simulink model "test_8m_0508"  (R2024a)
settings: Solver=FixedStepAuto  StartTime=0.0  StopTime=30  FixedStep=dt  RelTol=1e-3
values from neighbouring files (symbols this model uses):
  attitude_0 = [0; -90;  -0]    [ini_param_8m_0522.m]
  b = 4.0    (= 4)    [ini_param_8m_0522.m]
  cbar = 0.75    [ini_param_8m_0522.m]
  dt = 0.004    [ini_param_8m_0522.m]
  H = 1000    [ini_param_8m_0522.m]
  N_data = [0,200, 491, 804, 1077, 1344, 1559, 1832, 2078, 2318, 2579,            2864, 3117, 3371, 3608.2, 3872, 4055.7, 4291, 4507, 4739, 4935]'    [cal_motor.m]
  N_pwm = 0.01*[0, 5 ,10 ,15 ,20 ,25 ,30 ,35,40, 45 ,50 ,              55 ,60 ,65 ,70, 75, 80 , 85 ,90 ,95 ,100]'    [cal_motor.m]
  pitch_rate_K = 1    [ini_param_8m_0522.m]
  roll_rate_K = 1    [ini_param_8m_0522.m]
  S = 6.0    (= 6)    [ini_param_8m_0522.m]
  Ts = 0.05    [ini_param_8m_0522.m]
  Ts_sur = 0.25    [ini_param_8m_0522.m]
  yaw_rate_K = 1    [ini_param_8m_0522.m]
undefined symbols (not defined in the file or in its folder): sigbuilder_block, UAV
libraries: slpidlib x9, simulink_extras x6, sharedtransform x2, shared6dof x1
(part 3 of 11)

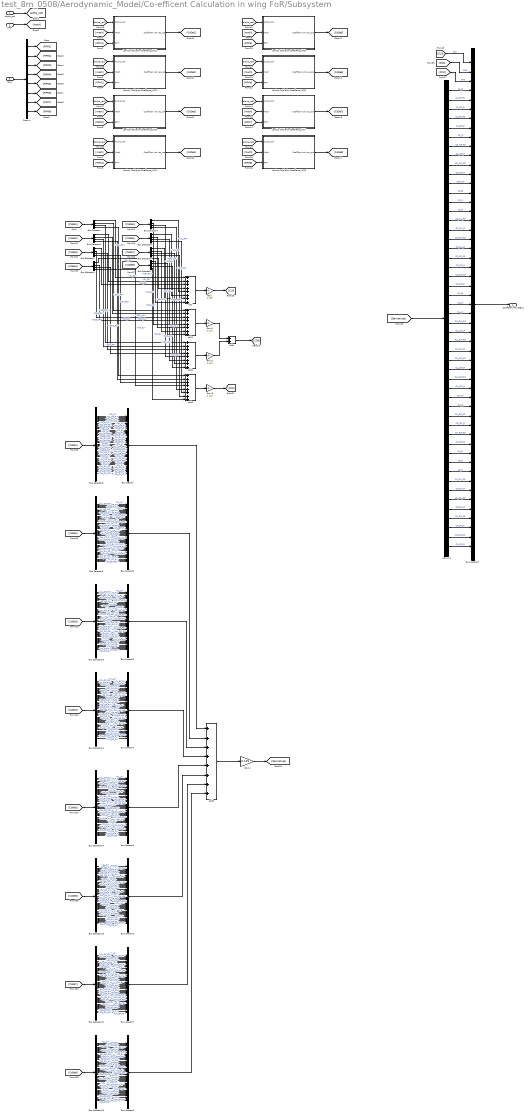
== system test_8m_0508/Aerodynamic_Model/Co-efficent Calculation in wing FoR/Subsystem ==
  alpha_rad : Inport
  Mach : Inport  Port=2
  RPM : Inport  Port=3
  Add{,1..3,5} (5 alike) : Sum  Inputs=++++++++
  Add4 : Sum
  Bus Creator{,2..8} (8 alike) : BusCreator  Inputs=50
  Bus Creator1 : BusCreator  Inputs=53
  Bus Selector : BusSelector  OutputSignals=CL_FR,CDI_FR,CD0_FR,CM_FR
  Bus Selector1 : BusSelector  OutputSignals=CL_FR,CDI_FR,CD0_FR,CM_FR
  Bus Selector{8..15} (8 alike) : BusSelector  OutputSignals=CL_Q,CL_DF_FO,CL_DF_FI,CL_DF_RO,CL_DF_RI,CD_Q,CD_DF_FO,CD_DF_FI,CD_DF_RO,CD_DF_RI,CD0_AF,CS_B,CS_P,CS_R,CS_DA_FO,CS_DA_FI,CS_DA_RO,CS_DA_RI,CS_DF_FO,CS_DF_FI,CS_DF_RO,CS_DF_RI,CLL_B,CLL_P,CLL_R,CLL_DA_FO,CLL_DA_FI,CLL_DA_RO,CLL_DA_RI,CLL_DF_FO,CLL_DF_FI,CLL_DF_RO,CLL_DF_RI,CM_AF,CM_Q,CM_DF_FO,CM_DF_FI,CM_DF_RO,CM_DF_RI,CN_B,CN_P,CN_R,CN_DA_FO,CN_DA_FI,CN_DA_RO,CN_DA_RI,CN_DF_FO,CN_DF_FI,CN_DF_RO,CN_DF_RI
  Bus Selector2 : BusSelector  OutputSignals=CL_FL,CDI_FL,CD0_FL,CM_FL
  Bus Selector3 : BusSelector  OutputSignals=CL_FL,CDI_FL,CD0_FL,CM_FL
  Bus Selector4 : BusSelector  OutputSignals=CL_RR,CDI_RR,CD0_RR,CM_RR
  Bus Selector5 : BusSelector  OutputSignals=CL_RR,CDI_RR,CD0_RR,CM_RR
  Bus Selector6 : BusSelector  OutputSignals=CL_RL,CDI_RL,CD0_RL,CM_RL
  Bus Selector7 : BusSelector  OutputSignals=CL_RL,CDI_RL,CD0_RL,CM_RL
  Demux : Demux  Outputs=8
  Demux1 : Demux  Outputs=50
  Gain{,1..4} (5 alike) : Gain  Gain=0.125
  LookUp Table for Coeffients_WS1 : Subsystem
  LookUp Table for Coeffients_WS2 : Subsystem
  LookUp Table for Coeffients_WS3 : Subsystem
  LookUp Table for Coeffients_WS4 : Subsystem
  LookUp Table for Coeffients_WS5 : Subsystem
  LookUp Table for Coeffients_WS6 : Subsystem
  LookUp Table for Coeffients_WS7 : Subsystem
  LookUp Table for Coeffients_WS8 : Subsystem
  CoeffDerivativesBus : Outport
  wires:
  [alpha_rad] -> LookUp Table for Coeffients_WS6/1(alpha_rad)
  [alpha_rad] -> LookUp Table for Coeffients_WS5/1(alpha_rad)
  [alpha_rad] -> LookUp Table for Coeffients_WS7/1(alpha_rad)
  [alpha_rad] -> LookUp Table for Coeffients_WS4/1(alpha_rad)
  [alpha_rad] -> LookUp Table for Coeffients_WS8/1(alpha_rad)
  [alpha_rad] -> LookUp Table for Coeffients_WS3/1(alpha_rad)
  [alpha_rad] -> LookUp Table for Coeffients_WS2/1(alpha_rad)
  [alpha_rad] -> LookUp Table for Coeffients_WS1/1(alpha_rad)
  RPM/1 -> Demux/1
  Demux/1 -> [RPM1]
  alpha_rad/1 -> [alpha_rad]
  Mach/1 -> [mach]
  Demux/2 -> [RPM2]
  Demux/3 -> [RPM3]
  Demux/4 -> [RPM4]
  Demux/5 -> [RPM5]
  Demux/6 -> [RPM6]
  Demux/7 -> [RPM7]
  Demux/8 -> [RPM8]
  [mach] -> LookUp Table for Coeffients_WS1/2(Mach)
  [RPM1] -> LookUp Table for Coeffients_WS1/3(RPM)
  [mach] -> LookUp Table for Coeffients_WS2/2(Mach)
  [RPM2] -> LookUp Table for Coeffients_WS2/3(RPM)
  [mach] -> LookUp Table for Coeffients_WS3/2(Mach)
  [RPM3] -> LookUp Table for Coeffients_WS3/3(RPM)
  [mach] -> LookUp Table for Coeffients_WS4/2(Mach)
  [RPM4] -> LookUp Table for Coeffients_WS4/3(RPM)
  [mach] -> LookUp Table for Coeffients_WS5/2(Mach)
  [RPM5] -> LookUp Table for Coeffients_WS5/3(RPM)
  [mach] -> LookUp Table for Coeffients_WS6/2(Mach)
  [RPM6] -> LookUp Table for Coeffients_WS6/3(RPM)
  [mach] -> LookUp Table for Coeffients_WS7/2(Mach)
  [RPM7] -> LookUp Table for Coeffients_WS7/3(RPM)
  [mach] -> LookUp Table for Coeffients_WS8/2(Mach)
  [RPM8] -> LookUp Table for Coeffients_WS8/3(RPM)
  LookUp Table for Coeffients_WS1/1(CoeffDerivatives_rad) -> [CoDe1]
  LookUp Table for Coeffients_WS2/1(CoeffDerivatives_rad) -> [CoDe2]
  LookUp Table for Coeffients_WS3/1(CoeffDerivatives_rad) -> [CoDe3]
  LookUp Table for Coeffients_WS4/1(CoeffDerivatives_rad) -> [CoDe4]
  LookUp Table for Coeffients_WS5/1(CoeffDerivatives_rad) -> [CoDe5]
  LookUp Table for Coeffients_WS6/1(CoeffDerivatives_rad) -> [CoDe6]
  LookUp Table for Coeffients_WS7/1(CoeffDerivatives_rad) -> [CoDe7]
  LookUp Table for Coeffients_WS8/1(CoeffDerivatives_rad) -> [CoDe8]
  Bus Creator1/1 -> CoeffDerivativesBus/1
  [CoDe1] -> Bus Selector/1
  [CoDe7] -> Bus Selector6/1
  [CoDe5] -> Bus Selector4/1
  [CoDe3] -> Bus Selector2/1
  [CoDe4] -> Bus Selector3/1
  [CoDe2] -> Bus Selector1/1
  [CoDe6] -> Bus Selector5/1
  [CoDe8] -> Bus Selector7/1
  Bus Selector/1 -> Add/1  "<CL_FR>"
  Bus Selector1/1 -> Add/2  "<CL_FR>"
  Bus Selector2/1 -> Add/3  "<CL_FL>"
  Bus Selector3/1 -> Add/4  "<CL_FL>"
  Bus Selector4/1 -> Add/5  "<CL_RR>"
  Bus Selector5/1 -> Add/6  "<CL_RR>"
  Bus Selector6/1 -> Add/7  "<CL_RL>"
  Bus Selector7/1 -> Add/8  "<CL_RL>"
  Add/1 -> Gain/1
  Add1/1 -> Gain1/1
  Add2/1 -> Gain2/1
  Add3/1 -> Gain3/1
  Bus Selector/2 -> Add1/1  "<CDI_FR>"
  Bus Selector1/2 -> Add1/2  "<CDI_FR>"
  Bus Selector2/2 -> Add1/3  "<CDI_FL>"
  Bus Selector3/2 -> Add1/4  "<CDI_FL>"
  Bus Selector4/2 -> Add1/5  "<CDI_RR>"
  Bus Selector5/2 -> Add1/6  "<CDI_RR>"
  Bus Selector6/2 -> Add1/7  "<CDI_RL>"
  Bus Selector7/2 -> Add1/8  "<CDI_RL>"
  Bus Selector/3 -> Add2/1  "<CD0_FR>"
  Bus Selector1/3 -> Add2/2  "<CD0_FR>"
  Bus Selector2/3 -> Add2/3  "<CD0_FL>"
  Bus Selector3/3 -> Add2/4  "<CD0_FL>"
  Bus Selector4/3 -> Add2/5  "<CD0_RR>"
  Bus Selector5/3 -> Add2/6  "<CD0_RR>"
  Bus Selector6/3 -> Add2/7  "<CD0_RL>"
  Bus Selector7/3 -> Add2/8  "<CD0_RL>"
  Bus Selector/4 -> Add3/1  "<CM_FR>"
  Bus Selector1/4 -> Add3/2  "<CM_FR>"
  Bus Selector2/4 -> Add3/3  "<CM_FL>"
  Bus Selector3/4 -> Add3/4  "<CM_FL>"
  Bus Selector4/4 -> Add3/5  "<CM_RR>"
  Bus Selector5/4 -> Add3/6  "<CM_RR>"
  Bus Selector6/4 -> Add3/7  "<CM_RL>"
  Bus Selector7/4 -> Add3/8  "<CM_RL>"
  Gain/1 -> [CL0]
  Gain1/1 -> Add4/1
  Gain2/1 -> Add4/2
  Gain3/1 -> [CM0]
  Add4/1 -> [CD0]
  [CoDe1] -> Bus Selector8/1
  Bus Selector8/1 -> Bus Creator/1  "<CL_Q>"
  Bus Selector8/2 -> Bus Creator/2  "<CL_DF_FO>"
  Bus Selector8/3 -> Bus Creator/3  "<CL_DF_FI>"
  Bus Selector8/4 -> Bus Creator/4  "<CL_DF_RO>"
  Bus Selector8/5 -> Bus Creator/5  "<CL_DF_RI>"
  Bus Selector8/6 -> Bus Creator/6  "<CD_Q>"
  Bus Selector8/7 -> Bus Creator/7  "<CD_DF_FO>"
  Bus Selector8/8 -> Bus Creator/8  "<CD_DF_FI>"
  Bus Selector8/9 -> Bus Creator/9  "<CD_DF_RO>"
  Bus Selector8/10 -> Bus Creator/10  "<CD_DF_RI>"
  Bus Selector8/11 -> Bus Creator/11  "<CD0_AF>"
  Bus Selector8/12 -> Bus Creator/12  "<CS_B>"
  Bus Selector8/13 -> Bus Creator/13  "<CS_P>"
  Bus Selector8/14 -> Bus Creator/14  "<CS_R>"
  Bus Selector8/15 -> Bus Creator/15  "<CS_DA_FO>"
  Bus Selector8/16 -> Bus Creator/16  "<CS_DA_FI>"
  Bus Selector8/17 -> Bus Creator/17  "<CS_DA_RO>"
  Bus Selector8/18 -> Bus Creator/18  "<CS_DA_RI>"
  Bus Selector8/19 -> Bus Creator/19  "<CS_DF_FO>"
  Bus Selector8/20 -> Bus Creator/20  "<CS_DF_FI>"
  Bus Selector8/21 -> Bus Creator/21  "<CS_DF_RO>"
  Bus Selector8/22 -> Bus Creator/22  "<CS_DF_RI>"
  Bus Selector8/23 -> Bus Creator/23  "<CLL_B>"
  Bus Selector8/24 -> Bus Creator/24  "<CLL_P>"
  Bus Selector8/25 -> Bus Creator/25  "<CLL_R>"
  Bus Selector8/26 -> Bus Creator/26  "<CLL_DA_FO>"
  Bus Selector8/27 -> Bus Creator/27  "<CLL_DA_FI>"
  Bus Selector8/28 -> Bus Creator/28  "<CLL_DA_RO>"
  Bus Selector8/29 -> Bus Creator/29  "<CLL_DA_RI>"
  Bus Selector8/30 -> Bus Creator/30  "<CLL_DF_FO>"
  Bus Selector8/31 -> Bus Creator/31  "<CLL_DF_FI>"
  Bus Selector8/32 -> Bus Creator/32  "<CLL_DF_RO>"
  Bus Selector8/33 -> Bus Creator/33  "<CLL_DF_RI>"
  Bus Selector8/34 -> Bus Creator/34  "<CM_AF>"
  Bus Selector8/35 -> Bus Creator/35  "<CM_Q>"
  Bus Selector8/36 -> Bus Creator/36  "<CM_DF_FO>"
  Bus Selector8/37 -> Bus Creator/37  "<CM_DF_FI>"
  Bus Selector8/38 -> Bus Creator/38  "<CM_DF_RO>"
  Bus Selector8/39 -> Bus Creator/39  "<CM_DF_RI>"
  Bus Selector8/40 -> Bus Creator/40  "<CN_B>"
  Bus Selector8/41 -> Bus Creator/41  "<CN_P>"
  Bus Selector8/42 -> Bus Creator/42  "<CN_R>"
  Bus Selector8/43 -> Bus Creator/43  "<CN_DA_FO>"
  Bus Selector8/44 -> Bus Creator/44  "<CN_DA_FI>"
  Bus Selector8/45 -> Bus Creator/45  "<CN_DA_RO>"
  Bus Selector8/46 -> Bus Creator/46  "<CN_DA_RI>"
  Bus Selector8/47 -> Bus Creator/47  "<CN_DF_FO>"
  Bus Selector8/48 -> Bus Creator/48  "<CN_DF_FI>"
  Bus Selector8/49 -> Bus Creator/49  "<CN_DF_RO>"
  Bus Selector8/50 -> Bus Creator/50  "<CN_DF_RI>"
  Bus Selector9/21 -> Bus Creator2/21  "<CS_DF_RO>"
  Bus Selector9/26 -> Bus Creator2/26  "<CLL_DA_FO>"
  Bus Selector9/19 -> Bus Creator2/19  "<CS_DF_FO>"
  Bus Selector9/22 -> Bus Creator2/22  "<CS_DF_RI>"
  Bus Selector9/16 -> Bus Creator2/16  "<CS_DA_FI>"
  Bus Selector9/13 -> Bus Creator2/13  "<CS_P>"
  Bus Selector9/17 -> Bus Creator2/17  "<CS_DA_RO>"
  Bus Selector9/14 -> Bus Creator2/14  "<CS_R>"
  Bus Selector9/15 -> Bus Creator2/15  "<CS_DA_FO>"
  Bus Selector9/12 -> Bus Creator2/12  "<CS_B>"
  Bus Selector9/18 -> Bus Creator2/18  "<CS_DA_RI>"
  Bus Selector9/8 -> Bus Creator2/8  "<CD_DF_FI>"
  Bus Selector9/7 -> Bus Creator2/7  "<CD_DF_FO>"
  Bus Selector9/9 -> Bus Creator2/9  "<CD_DF_RO>"
  Bus Selector9/3 -> Bus Creator2/3  "<CL_DF_FI>"
  Bus Selector9/4 -> Bus Creator2/4  "<CL_DF_RO>"
  Bus Selector9/5 -> Bus Creator2/5  "<CL_DF_RI>"
  Bus Selector9/28 -> Bus Creator2/28  "<CLL_DA_RO>"
  [CoDe2] -> Bus Selector9/1
  Bus Selector9/40 -> Bus Creator2/40  "<CN_B>"
  Bus Selector9/27 -> Bus Creator2/27  "<CLL_DA_FI>"
  Bus Selector9/39 -> Bus Creator2/39  "<CM_DF_RI>"
  Bus Selector9/24 -> Bus Creator2/24  "<CLL_P>"
  Bus Selector9/33 -> Bus Creator2/33  "<CLL_DF_RI>"
  Bus Selector9/31 -> Bus Creator2/31  "<CLL_DF_FI>"
  Bus Selector9/32 -> Bus Creator2/32  "<CLL_DF_RO>"
  Bus Selector9/37 -> Bus Creator2/37  "<CM_DF_FI>"
  Bus Selector9/35 -> Bus Creator2/35  "<CM_Q>"
  Bus Selector9/34 -> Bus Creator2/34  "<CM_AF>"
  Bus Selector9/38 -> Bus Creator2/38  "<CM_DF_RO>"
  Bus Selector9/11 -> Bus Creator2/11  "<CD0_AF>"
  Bus Selector9/36 -> Bus Creator2/36  "<CM_DF_FO>"
  Bus Selector9/30 -> Bus Creator2/30  "<CLL_DF_FO>"
  Bus Selector9/29 -> Bus Creator2/29  "<CLL_DA_RI>"
  Bus Selector9/6 -> Bus Creator2/6  "<CD_Q>"
  Bus Selector9/49 -> Bus Creator2/49  "<CN_DF_RO>"
  Bus Selector9/23 -> Bus Creator2/23  "<CLL_B>"
  Bus Selector9/50 -> Bus Creator2/50  "<CN_DF_RI>"
  Bus Selector9/20 -> Bus Creator2/20  "<CS_DF_FI>"
  Bus Selector9/48 -> Bus Creator2/48  "<CN_DF_FI>"
  Bus Selector9/47 -> Bus Creator2/47  "<CN_DF_FO>"
  Bus Selector9/44 -> Bus Creator2/44  "<CN_DA_FI>"
  Bus Selector9/42 -> Bus Creator2/42  "<CN_R>"
  Bus Selector9/10 -> Bus Creator2/10  "<CD_DF_RI>"
  Bus Selector9/25 -> Bus Creator2/25  "<CLL_R>"
  Bus Selector9/45 -> Bus Creator2/45  "<CN_DA_RO>"
  Bus Selector9/43 -> Bus Creator2/43  "<CN_DA_FO>"
  Bus Selector9/46 -> Bus Creator2/46  "<CN_DA_RI>"
  Bus Selector9/2 -> Bus Creator2/2  "<CL_DF_FO>"
  Bus Selector9/41 -> Bus Creator2/41  "<CN_P>"
  Bus Selector9/1 -> Bus Creator2/1  "<CL_Q>"
  Bus Selector11/9 -> Bus Creator4/9  "<CD_DF_RO>"
  Bus Selector11/7 -> Bus Creator4/7  "<CD_DF_FO>"
  Bus Selector11/14 -> Bus Creator4/14  "<CS_R>"
  Bus Selector11/17 -> Bus Creator4/17  "<CS_DA_RO>"
  Bus Selector11/8 -> Bus Creator4/8  "<CD_DF_FI>"
  Bus Selector11/12 -> Bus Creator4/12  "<CS_B>"
  Bus Selector11/15 -> Bus Creator4/15  "<CS_DA_FO>"
  Bus Selector11/19 -> Bus Creator4/19  "<CS_DF_FO>"
  Bus Selector11/26 -> Bus Creator4/26  "<CLL_DA_FO>"
  Bus Selector11/13 -> Bus Creator4/13  "<CS_P>"
  Bus Selector11/16 -> Bus Creator4/16  "<CS_DA_FI>"
  Bus Selector11/21 -> Bus Creator4/21  "<CS_DF_RO>"
  Bus Selector10/28 -> Bus Creator3/28  "<CLL_DA_RO>"
  Bus Selector10/27 -> Bus Creator3/27  "<CLL_DA_FI>"
  Bus Selector10/23 -> Bus Creator3/23  "<CLL_B>"
  Bus Selector10/25 -> Bus Creator3/25  "<CLL_R>"
  Bus Selector10/20 -> Bus Creator3/20  "<CS_DF_FI>"
  Bus Selector10/21 -> Bus Creator3/21  "<CS_DF_RO>"
  Bus Selector10/26 -> Bus Creator3/26  "<CLL_DA_FO>"
  Bus Selector10/24 -> Bus Creator3/24  "<CLL_P>"
  Bus Selector10/19 -> Bus Creator3/19  "<CS_DF_FO>"
  Bus Selector10/22 -> Bus Creator3/22  "<CS_DF_RI>"
  Bus Selector10/16 -> Bus Creator3/16  "<CS_DA_FI>"
  Bus Selector10/13 -> Bus Creator3/13  "<CS_P>"
  Bus Selector10/17 -> Bus Creator3/17  "<CS_DA_RO>"
  Bus Selector10/14 -> Bus Creator3/14  "<CS_R>"
  Bus Selector10/15 -> Bus Creator3/15  "<CS_DA_FO>"
  Bus Selector10/11 -> Bus Creator3/11  "<CD0_AF>"
  Bus Selector10/10 -> Bus Creator3/10  "<CD_DF_RI>"
  Bus Selector10/12 -> Bus Creator3/12  "<CS_B>"
  Bus Selector10/18 -> Bus Creator3/18  "<CS_DA_RI>"
  Bus Selector10/8 -> Bus Creator3/8  "<CD_DF_FI>"
  Bus Selector10/7 -> Bus Creator3/7  "<CD_DF_FO>"
  Bus Selector10/9 -> Bus Creator3/9  "<CD_DF_RO>"
  Bus Selector10/3 -> Bus Creator3/3  "<CL_DF_FI>"
  Bus Selector10/4 -> Bus Creator3/4  "<CL_DF_RO>"
  [CoDe3] -> Bus Selector10/1
  Bus Selector10/39 -> Bus Creator3/39  "<CM_DF_RI>"
  Bus Selector10/37 -> Bus Creator3/37  "<CM_DF_FI>"
  Bus Selector10/34 -> Bus Creator3/34  "<CM_AF>"
  Bus Selector10/38 -> Bus Creator3/38  "<CM_DF_RO>"
  Bus Selector10/36 -> Bus Creator3/36  "<CM_DF_FO>"
  Bus Selector10/49 -> Bus Creator3/49  "<CN_DF_RO>"
  Bus Selector10/45 -> Bus Creator3/45  "<CN_DA_RO>"
  Bus Selector10/46 -> Bus Creator3/46  "<CN_DA_RI>"
  Bus Selector10/42 -> Bus Creator3/42  "<CN_R>"
  Bus Selector10/41 -> Bus Creator3/41  "<CN_P>"
  Bus Selector10/43 -> Bus Creator3/43  "<CN_DA_FO>"
  Bus Selector10/29 -> Bus Creator3/29  "<CLL_DA_RI>"
  Bus Selector10/6 -> Bus Creator3/6  "<CD_Q>"
  Bus Selector11/1 -> Bus Creator4/1  "<CL_Q>"
  Bus Selector11/46 -> Bus Creator4/46  "<CN_DA_RI>"
  Bus Selector10/2 -> Bus Creator3/2  "<CL_DF_FO>"
  Bus Selector10/31 -> Bus Creator3/31  "<CLL_DF_FI>"
  Bus Selector11/41 -> Bus Creator4/41  "<CN_P>"
  Bus Selector11/25 -> Bus Creator4/25  "<CLL_R>"
  Bus Selector11/45 -> Bus Creator4/45  "<CN_DA_RO>"
  Bus Selector11/10 -> Bus Creator4/10  "<CD_DF_RI>"
  Bus Selector11/18 -> Bus Creator4/18  "<CS_DA_RI>"
  Bus Selector11/42 -> Bus Creator4/42  "<CN_R>"
  Bus Selector11/50 -> Bus Creator4/50  "<CN_DF_RI>"
  Bus Selector10/47 -> Bus Creator3/47  "<CN_DF_FO>"
  Bus Selector11/23 -> Bus Creator4/23  "<CLL_B>"
  Bus Selector11/48 -> Bus Creator4/48  "<CN_DF_FI>"
  Bus Selector11/20 -> Bus Creator4/20  "<CS_DF_FI>"
  Bus Selector10/50 -> Bus Creator3/50  "<CN_DF_RI>"
  Bus Selector11/6 -> Bus Creator4/6  "<CD_Q>"
  Bus Selector11/47 -> Bus Creator4/47  "<CN_DF_FO>"
  Bus Selector11/11 -> Bus Creator4/11  "<CD0_AF>"
  Bus Selector11/38 -> Bus Creator4/38  "<CM_DF_RO>"
  Bus Selector10/33 -> Bus Creator3/33  "<CLL_DF_RI>"
  Bus Selector11/30 -> Bus Creator4/30  "<CLL_DF_FO>"
  Bus Selector11/36 -> Bus Creator4/36  "<CM_DF_FO>"
  Bus Selector11/22 -> Bus Creator4/22  "<CS_DF_RI>"
  Bus Selector10/44 -> Bus Creator3/44  "<CN_DA_FI>"
  Bus Selector11/35 -> Bus Creator4/35  "<CM_Q>"
  Bus Selector10/35 -> Bus Creator3/35  "<CM_Q>"
  Bus Selector11/34 -> Bus Creator4/34  "<CM_AF>"
  Bus Selector10/32 -> Bus Creator3/32  "<CLL_DF_RO>"
  Bus Selector11/31 -> Bus Creator4/31  "<CLL_DF_FI>"
  Bus Selector11/2 -> Bus Creator4/2  "<CL_DF_FO>"
  Bus Selector11/40 -> Bus Creator4/40  "<CN_B>"
  Bus Selector11/24 -> Bus Creator4/24  "<CLL_P>"
  Bus Selector11/43 -> Bus Creator4/43  "<CN_DA_FO>"
  Bus Selector11/27 -> Bus Creator4/27  "<CLL_DA_FI>"
  Bus Selector10/30 -> Bus Creator3/30  "<CLL_DF_FO>"
  Bus Selector11/3 -> Bus Creator4/3  "<CL_DF_FI>"
  Bus Selector10/40 -> Bus Creator3/40  "<CN_B>"
  Bus Selector11/37 -> Bus Creator4/37  "<CM_DF_FI>"
  Bus Selector11/29 -> Bus Creator4/29  "<CLL_DA_RI>"
  Bus Selector11/5 -> Bus Creator4/5  "<CL_DF_RI>"
  [CoDe4] -> Bus Selector11/1
  Bus Selector11/33 -> Bus Creator4/33  "<CLL_DF_RI>"
  Bus Selector11/44 -> Bus Creator4/44  "<CN_DA_FI>"
  Bus Selector11/4 -> Bus Creator4/4  "<CL_DF_RO>"
  Bus Selector11/49 -> Bus Creator4/49  "<CN_DF_RO>"
  Bus Selector10/48 -> Bus Creator3/48  "<CN_DF_FI>"
  Bus Selector11/28 -> Bus Creator4/28  "<CLL_DA_RO>"
  Bus Selector10/1 -> Bus Creator3/1  "<CL_Q>"
  Bus Selector11/32 -> Bus Creator4/32  "<CLL_DF_RO>"
  Bus Selector11/39 -> Bus Creator4/39  "<CM_DF_RI>"
  Bus Selector10/5 -> Bus Creator3/5  "<CL_DF_RI>"
  Bus Selector12/19 -> Bus Creator7/19  "<CS_DF_FO>"
  Bus Selector12/22 -> Bus Creator7/22  "<CS_DF_RI>"
  Bus Selector12/27 -> Bus Creator7/27  "<CLL_DA_FI>"
  Bus Selector12/21 -> Bus Creator7/21  "<CS_DF_RO>"
  Bus Selector13/21 -> Bus Creator8/21  "<CS_DF_RO>"
  Bus Selector12/20 -> Bus Creator7/20  "<CS_DF_FI>"
  Bus Selector12/26 -> Bus Creator7/26  "<CLL_DA_FO>"
  Bus Selector12/25 -> Bus Creator7/25  "<CLL_R>"
  Bus Selector13/8 -> Bus Creator8/8  "<CD_DF_FI>"
  Bus Selector13/19 -> Bus Creator8/19  "<CS_DF_FO>"
  Bus Selector13/17 -> Bus Creator8/17  "<CS_DA_RO>"
  Bus Selector13/7 -> Bus Creator8/7  "<CD_DF_FO>"
  Bus Selector13/26 -> Bus Creator8/26  "<CLL_DA_FO>"
  Bus Selector13/13 -> Bus Creator8/13  "<CS_P>"
  Bus Selector13/9 -> Bus Creator8/9  "<CD_DF_RO>"
  Bus Selector15/9 -> Bus Creator6/9  "<CD_DF_RO>"
  Bus Selector15/7 -> Bus Creator6/7  "<CD_DF_FO>"
  Bus Selector15/14 -> Bus Creator6/14  "<CS_R>"
  Bus Selector12/24 -> Bus Creator7/24  "<CLL_P>"
  Bus Selector15/17 -> Bus Creator6/17  "<CS_DA_RO>"
  Bus Selector15/12 -> Bus Creator6/12  "<CS_B>"
  Bus Selector15/15 -> Bus Creator6/15  "<CS_DA_FO>"
  Bus Selector15/19 -> Bus Creator6/19  "<CS_DF_FO>"
  Bus Selector15/26 -> Bus Creator6/26  "<CLL_DA_FO>"
  Bus Selector15/13 -> Bus Creator6/13  "<CS_P>"
  Bus Selector15/16 -> Bus Creator6/16  "<CS_DA_FI>"
  Bus Selector15/21 -> Bus Creator6/21  "<CS_DF_RO>"
  Bus Selector14/28 -> Bus Creator5/28  "<CLL_DA_RO>"
  Bus Selector14/27 -> Bus Creator5/27  "<CLL_DA_FI>"
  Bus Selector14/23 -> Bus Creator5/23  "<CLL_B>"
  Bus Selector14/25 -> Bus Creator5/25  "<CLL_R>"
  Bus Selector14/26 -> Bus Creator5/26  "<CLL_DA_FO>"
  Bus Selector14/24 -> Bus Creator5/24  "<CLL_P>"
  Bus Selector14/19 -> Bus Creator5/19  "<CS_DF_FO>"
  Bus Selector14/22 -> Bus Creator5/22  "<CS_DF_RI>"
  Bus Selector14/16 -> Bus Creator5/16  "<CS_DA_FI>"
  Bus Selector14/13 -> Bus Creator5/13  "<CS_P>"
  Bus Selector14/15 -> Bus Creator5/15  "<CS_DA_FO>"
  Bus Selector14/11 -> Bus Creator5/11  "<CD0_AF>"
  Bus Selector14/10 -> Bus Creator5/10  "<CD_DF_RI>"
  Bus Selector14/12 -> Bus Creator5/12  "<CS_B>"
  Bus Selector14/18 -> Bus Creator5/18  "<CS_DA_RI>"
  Bus Selector14/8 -> Bus Creator5/8  "<CD_DF_FI>"
  Bus Selector14/7 -> Bus Creator5/7  "<CD_DF_FO>"
  Bus Selector14/9 -> Bus Creator5/9  "<CD_DF_RO>"
  Bus Selector14/3 -> Bus Creator5/3  "<CL_DF_FI>"
  Bus Selector13/15 -> Bus Creator8/15  "<CS_DA_FO>"
  Bus Selector14/4 -> Bus Creator5/4  "<CL_DF_RO>"
  Bus Selector14/5 -> Bus Creator5/5  "<CL_DF_RI>"
  Bus Selector12/1 -> Bus Creator7/1  "<CL_Q>"
  Bus Selector13/32 -> Bus Creator8/32  "<CLL_DF_RO>"
  Bus Selector14/17 -> Bus Creator5/17  "<CS_DA_RO>"
  Bus Selector12/5 -> Bus Creator7/5  "<CL_DF_RI>"
  Bus Selector13/49 -> Bus Creator8/49  "<CN_DF_RO>"
  Bus Selector13/4 -> Bus Creator8/4  "<CL_DF_RO>"
  Bus Selector13/33 -> Bus Creator8/33  "<CLL_DF_RI>"
  Bus Selector12/30 -> Bus Creator7/30  "<CLL_DF_FO>"
  Bus Selector13/5 -> Bus Creator8/5  "<CL_DF_RI>"
  Bus Selector14/20 -> Bus Creator5/20  "<CS_DF_FI>"
  [CoDe8] -> Bus Selector13/1
  Bus Selector14/21 -> Bus Creator5/21  "<CS_DF_RO>"
  Bus Selector12/40 -> Bus Creator7/40  "<CN_B>"
  Bus Selector13/37 -> Bus Creator8/37  "<CM_DF_FI>"
  Bus Selector13/3 -> Bus Creator8/3  "<CL_DF_FI>"
  Bus Selector13/44 -> Bus Creator8/44  "<CN_DA_FI>"
  Bus Selector13/24 -> Bus Creator8/24  "<CLL_P>"
  Bus Selector13/2 -> Bus Creator8/2  "<CL_DF_FO>"
  Bus Selector13/40 -> Bus Creator8/40  "<CN_B>"
  Bus Selector13/27 -> Bus Creator8/27  "<CLL_DA_FI>"
  Bus Selector13/31 -> Bus Creator8/31  "<CLL_DF_FI>"
  Bus Selector12/32 -> Bus Creator7/32  "<CLL_DF_RO>"
  Bus Selector13/34 -> Bus Creator8/34  "<CM_AF>"
  Bus Selector13/35 -> Bus Creator8/35  "<CM_Q>"
  Bus Selector12/35 -> Bus Creator7/35  "<CM_Q>"
  [CoDe5] -> Bus Selector14/1
  Bus Selector14/40 -> Bus Creator5/40  "<CN_B>"
  Bus Selector14/39 -> Bus Creator5/39  "<CM_DF_RI>"
  Bus Selector14/38 -> Bus Creator5/38  "<CM_DF_RO>"
  Bus Selector14/33 -> Bus Creator5/33  "<CLL_DF_RI>"
  Bus Selector14/32 -> Bus Creator5/32  "<CLL_DF_RO>"
  Bus Selector14/37 -> Bus Creator5/37  "<CM_DF_FI>"
  Bus Selector14/35 -> Bus Creator5/35  "<CM_Q>"
  Bus Selector14/34 -> Bus Creator5/34  "<CM_AF>"
  Bus Selector14/36 -> Bus Creator5/36  "<CM_DF_FO>"
  Bus Selector14/30 -> Bus Creator5/30  "<CLL_DF_FO>"
  Bus Selector14/29 -> Bus Creator5/29  "<CLL_DA_RI>"
  Bus Selector14/49 -> Bus Creator5/49  "<CN_DF_RO>"
  Bus Selector14/50 -> Bus Creator5/50  "<CN_DF_RI>"
  Bus Selector14/48 -> Bus Creator5/48  "<CN_DF_FI>"
  Bus Selector14/47 -> Bus Creator5/47  "<CN_DF_FO>"
  Bus Selector14/45 -> Bus Creator5/45  "<CN_DA_RO>"
  Bus Selector14/46 -> Bus Creator5/46  "<CN_DA_RI>"
  Bus Selector14/44 -> Bus Creator5/44  "<CN_DA_FI>"
  Bus Selector14/42 -> Bus Creator5/42  "<CN_R>"
  Bus Selector14/41 -> Bus Creator5/41  "<CN_P>"
  Bus Selector14/43 -> Bus Creator5/43  "<CN_DA_FO>"
  Bus Selector14/2 -> Bus Creator5/2  "<CL_DF_FO>"
  Bus Selector15/2 -> Bus Creator6/2  "<CL_DF_FO>"
  Bus Selector12/28 -> Bus Creator7/28  "<CLL_DA_RO>"
  Bus Selector15/43 -> Bus Creator6/43  "<CN_DA_FO>"
  Bus Selector15/46 -> Bus Creator6/46  "<CN_DA_RI>"
  Bus Selector15/41 -> Bus Creator6/41  "<CN_P>"
  Bus Selector14/31 -> Bus Creator5/31  "<CLL_DF_FI>"
  Bus Selector13/29 -> Bus Creator8/29  "<CLL_DA_RI>"
  Bus Selector15/45 -> Bus Creator6/45  "<CN_DA_RO>"
  Bus Selector15/44 -> Bus Creator6/44  "<CN_DA_FI>"
  Bus Selector15/25 -> Bus Creator6/25  "<CLL_R>"
  Bus Selector15/10 -> Bus Creator6/10  "<CD_DF_RI>"
  Bus Selector15/18 -> Bus Creator6/18  "<CS_DA_RI>"
  Bus Selector15/50 -> Bus Creator6/50  "<CN_DF_RI>"
  Bus Selector15/23 -> Bus Creator6/23  "<CLL_B>"
  Bus Selector15/20 -> Bus Creator6/20  "<CS_DF_FI>"
  Bus Selector15/49 -> Bus Creator6/49  "<CN_DF_RO>"
  Bus Selector12/23 -> Bus Creator7/23  "<CLL_B>"
  Bus Selector15/6 -> Bus Creator6/6  "<CD_Q>"
  Bus Selector15/11 -> Bus Creator6/11  "<CD0_AF>"
  Bus Selector15/47 -> Bus Creator6/47  "<CN_DF_FO>"
  Bus Selector15/38 -> Bus Creator6/38  "<CM_DF_RO>"
  Bus Selector15/30 -> Bus Creator6/30  "<CLL_DF_FO>"
  Bus Selector15/36 -> Bus Creator6/36  "<CM_DF_FO>"
  Bus Selector15/22 -> Bus Creator6/22  "<CS_DF_RI>"
  Bus Selector15/35 -> Bus Creator6/35  "<CM_Q>"
  Bus Selector13/12 -> Bus Creator8/12  "<CS_B>"
  Bus Selector15/34 -> Bus Creator6/34  "<CM_AF>"
  Bus Selector15/37 -> Bus Creator6/37  "<CM_DF_FI>"
  Bus Selector13/39 -> Bus Creator8/39  "<CM_DF_RI>"
  Bus Selector15/31 -> Bus Creator6/31  "<CLL_DF_FI>"
  Bus Selector15/32 -> Bus Creator6/32  "<CLL_DF_RO>"
  Bus Selector15/24 -> Bus Creator6/24  "<CLL_P>"
  Bus Selector15/27 -> Bus Creator6/27  "<CLL_DA_FI>"
  Bus Selector15/3 -> Bus Creator6/3  "<CL_DF_FI>"
  Bus Selector15/4 -> Bus Creator6/4  "<CL_DF_RO>"
  Bus Selector13/43 -> Bus Creator8/43  "<CN_DA_FO>"
  Bus Selector12/2 -> Bus Creator7/2  "<CL_DF_FO>"
  Bus Selector13/14 -> Bus Creator8/14  "<CS_R>"
  Bus Selector12/31 -> Bus Creator7/31  "<CLL_DF_FI>"
  Bus Selector12/6 -> Bus Creator7/6  "<CD_Q>"
  Bus Selector12/46 -> Bus Creator7/46  "<CN_DA_RI>"
  Bus Selector12/43 -> Bus Creator7/43  "<CN_DA_FO>"
  Bus Selector12/42 -> Bus Creator7/42  "<CN_R>"
  Bus Selector15/28 -> Bus Creator6/28  "<CLL_DA_RO>"
  Bus Selector13/46 -> Bus Creator8/46  "<CN_DA_RI>"
  Bus Selector12/41 -> Bus Creator7/41  "<CN_P>"
  Bus Selector13/45 -> Bus Creator8/45  "<CN_DA_RO>"
  Bus Selector12/38 -> Bus Creator7/38  "<CM_DF_RO>"
  Bus Selector12/39 -> Bus Creator7/39  "<CM_DF_RI>"
  [CoDe7] -> Bus Selector12/1
  Bus Selector15/42 -> Bus Creator6/42  "<CN_R>"
  Bus Selector12/34 -> Bus Creator7/34  "<CM_AF>"
  Bus Selector12/37 -> Bus Creator7/37  "<CM_DF_FI>"
  Bus Selector12/45 -> Bus Creator7/45  "<CN_DA_RO>"
  Bus Selector13/28 -> Bus Creator8/28  "<CLL_DA_RO>"
  Bus Selector12/15 -> Bus Creator7/15  "<CS_DA_FO>"
  Bus Selector12/12 -> Bus Creator7/12  "<CS_B>"
  Bus Selector12/48 -> Bus Creator7/48  "<CN_DF_FI>"
  Bus Selector12/11 -> Bus Creator7/11  "<CD0_AF>"
  Bus Selector12/14 -> Bus Creator7/14  "<CS_R>"
  Bus Selector12/29 -> Bus Creator7/29  "<CLL_DA_RI>"
  Bus Selector12/7 -> Bus Creator7/7  "<CD_DF_FO>"
  [CoDe6] -> Bus Selector15/1
  Bus Selector12/8 -> Bus Creator7/8  "<CD_DF_FI>"
  Bus Selector12/3 -> Bus Creator7/3  "<CL_DF_FI>"
  Bus Selector15/5 -> Bus Creator6/5  "<CL_DF_RI>"
  Bus Selector15/29 -> Bus Creator6/29  "<CLL_DA_RI>"
  Bus Selector12/10 -> Bus Creator7/10  "<CD_DF_RI>"
  Bus Selector12/18 -> Bus Creator7/18  "<CS_DA_RI>"
  Bus Selector12/17 -> Bus Creator7/17  "<CS_DA_RO>"
  Bus Selector12/13 -> Bus Creator7/13  "<CS_P>"
  Bus Selector14/14 -> Bus Creator5/14  "<CS_R>"
  Bus Selector13/25 -> Bus Creator8/25  "<CLL_R>"
  Bus Selector12/44 -> Bus Creator7/44  "<CN_DA_FI>"
  Bus Selector12/49 -> Bus Creator7/49  "<CN_DF_RO>"
  Bus Selector13/36 -> Bus Creator8/36  "<CM_DF_FO>"
  Bus Selector15/1 -> Bus Creator6/1  "<CL_Q>"
  Bus Selector14/6 -> Bus Creator5/6  "<CD_Q>"
  Bus Selector13/22 -> Bus Creator8/22  "<CS_DF_RI>"
  Bus Selector13/41 -> Bus Creator8/41  "<CN_P>"
  Bus Selector13/30 -> Bus Creator8/30  "<CLL_DF_FO>"
  Bus Selector13/1 -> Bus Creator8/1  "<CL_Q>"
  Bus Selector12/33 -> Bus Creator7/33  "<CLL_DF_RI>"
  Bus Selector15/33 -> Bus Creator6/33  "<CLL_DF_RI>"
  Bus Selector13/11 -> Bus Creator8/11  "<CD0_AF>"
  Bus Selector13/6 -> Bus Creator8/6  "<CD_Q>"
  Bus Selector12/9 -> Bus Creator7/9  "<CD_DF_RO>"
  Bus Selector15/40 -> Bus Creator6/40  "<CN_B>"
  Bus Selector13/38 -> Bus Creator8/38  "<CM_DF_RO>"
  Bus Selector13/47 -> Bus Creator8/47  "<CN_DF_FO>"
  Bus Selector13/20 -> Bus Creator8/20  "<CS_DF_FI>"
  Bus Selector15/8 -> Bus Creator6/8  "<CD_DF_FI>"
  Bus Selector13/50 -> Bus Creator8/50  "<CN_DF_RI>"
  Bus Selector15/48 -> Bus Creator6/48  "<CN_DF_FI>"
  Bus Selector12/36 -> Bus Creator7/36  "<CM_DF_FO>"
  Bus Selector12/16 -> Bus Creator7/16  "<CS_DA_FI>"
  Bus Selector13/10 -> Bus Creator8/10  "<CD_DF_RI>"
  Bus Selector13/18 -> Bus Creator8/18  "<CS_DA_RI>"
  Bus Selector12/4 -> Bus Creator7/4  "<CL_DF_RO>"
  Bus Selector12/47 -> Bus Creator7/47  "<CN_DF_FO>"
  Bus Selector13/42 -> Bus Creator8/42  "<CN_R>"
  Bus Selector13/16 -> Bus Creator8/16  "<CS_DA_FI>"
  Bus Selector12/50 -> Bus Creator7/50  "<CN_DF_RI>"
  Bus Selector13/48 -> Bus Creator8/48  "<CN_DF_FI>"
  Bus Selector15/39 -> Bus Creator6/39  "<CM_DF_RI>"
  Bus Selector13/23 -> Bus Creator8/23  "<CLL_B>"
  Bus Selector14/1 -> Bus Creator5/1  "<CL_Q>"
  [CL0] -> Bus Creator1/1  "CL0"
  [CD0] -> Bus Creator1/2  "CD0"
  [CM0] -> Bus Creator1/3  "CM0"
  Demux1/1 -> Bus Creator1/4  "CL_Q"
  Demux1/2 -> Bus Creator1/5  "CL_DF_FO"
  Add5/1 -> Gain4/1
  Bus Creator/1 -> Add5/1
  Bus Creator2/1 -> Add5/2
  Bus Creator3/1 -> Add5/3
  Bus Creator4/1 -> Add5/4
  Bus Creator5/1 -> Add5/5
  Bus Creator6/1 -> Add5/6
  Bus Creator7/1 -> Add5/7
  Bus Creator8/1 -> Add5/8
  Gain4/1 -> [Derivatives]
  [Derivatives] -> Demux1/1
  Demux1/3 -> Bus Creator1/6  "CL_DF_FI"
  Demux1/4 -> Bus Creator1/7  "CL_DF_RO"
  Demux1/5 -> Bus Creator1/8  "CL_DF_RI"
  Demux1/6 -> Bus Creator1/9  "CD_Q"
  Demux1/7 -> Bus Creator1/10  "CD_DF_FO"
  Demux1/8 -> Bus Creator1/11  "CD_DF_FI"
  Demux1/9 -> Bus Creator1/12  "CD_DF_RO"
  Demux1/10 -> Bus Creator1/13  "CD_DF_RI"
  Demux1/11 -> Bus Creator1/14  "CD0_AF"
  Demux1/12 -> Bus Creator1/15  "CS_B"
  Demux1/13 -> Bus Creator1/16  "CS_P"
  Demux1/14 -> Bus Creator1/17  "CS_R"
  Demux1/15 -> Bus Creator1/18  "CS_DA_FO"
  Demux1/16 -> Bus Creator1/19  "CS_DA_FI"
  Demux1/17 -> Bus Creator1/20  "CS_DA_RO"
  Demux1/18 -> Bus Creator1/21  "CS_DA_RI"
  Demux1/19 -> Bus Creator1/22  "CS_DF_FO"
  Demux1/20 -> Bus Creator1/23  "CS_DF_FI"
  Demux1/21 -> Bus Creator1/24  "CS_DF_RO"
  Demux1/22 -> Bus Creator1/25  "CS_DF_RI"
  Demux1/23 -> Bus Creator1/26  "CLL_B"
  Demux1/24 -> Bus Creator1/27  "CLL_P"
  Demux1/25 -> Bus Creator1/28  "CLL_R"
  Demux1/26 -> Bus Creator1/29  "CLL_DA_FO"
  Demux1/27 -> Bus Creator1/30  "CLL_DA_FI"
  Demux1/28 -> Bus Creator1/31  "CLL_DA_RO"
  Demux1/29 -> Bus Creator1/32  "CLL_DA_RI"
  Demux1/30 -> Bus Creator1/33  "CLL_DF_FO"
  Demux1/31 -> Bus Creator1/34  "CLL_DF_FI"
  Demux1/32 -> Bus Creator1/35  "CLL_DF_RO"
  Demux1/33 -> Bus Creator1/36  "CLL_DF_RI"
  Demux1/34 -> Bus Creator1/37  "CM_AF"
  Demux1/35 -> Bus Creator1/38  "CM_Q"
  Demux1/36 -> Bus Creator1/39  "CM_DF_FO"
  Demux1/37 -> Bus Creator1/40  "CM_DF_FI"
  Demux1/38 -> Bus Creator1/41  "CM_DF_RO"
  Demux1/39 -> Bus Creator1/42  "CM_DF_RI"
  Demux1/40 -> Bus Creator1/43  "CN_B"
  Demux1/41 -> Bus Creator1/44  "CN_P"
  Demux1/42 -> Bus Creator1/45  "CN_R"
  Demux1/43 -> Bus Creator1/46  "CN_DA_FO"
  Demux1/44 -> Bus Creator1/47  "CN_DA_FI"
  Demux1/45 -> Bus Creator1/48  "CN_DA_RO"
  Demux1/46 -> Bus Creator1/49  "CN_DA_RI"
  Demux1/47 -> Bus Creator1/50  "CN_DF_FO"
  Demux1/48 -> Bus Creator1/51  "CN_DF_FI"
  Demux1/49 -> Bus Creator1/52  "CN_DF_RO"
  Demux1/50 -> Bus Creator1/53  "CN_DF_RI"

== system test_8m_0508/Aerodynamic_Model/Co-efficent Calculation in wing FoR/body2wing FoR ==
  u_body : Inport
  w_body : Inport  Port=2
  Add : Sum
  Add1 : Sum
  Cos2 : Trigonometry  Operator=cos
  Gain2 : Gain  Gain=-1
  Product{,1..3} (4 alike) : Product
  Sin2 : Trigonometry
  body_wing_angle : Constant  Value=45*pi/180
  u_wing : Outport
  w_wing : Outport  Port=2
  wires:
  Cos2/1 -> [cosGamm]
  Sin2/1 -> [sinGamm]
  [sinGamm] -> Gain2/1
  body_wing_angle/1 -> Sin2/1, Cos2/1
  [cosGamm] -> Product/2
  u_body/1 -> Product1/1, Product/1
  [sinGamm] -> Product1/2
  w_body/1 -> Product3/1, Product2/1
  Gain2/1 -> Product2/2
  [cosGamm] -> Product3/2
  Product/1 -> Add/1
  Product2/1 -> Add/2
  Product1/1 -> Add1/1
  Product3/1 -> Add1/2
  Add/1 -> u_wing/1
  Add1/1 -> w_wing/1

== system test_8m_0508/Aerodynamic_Model/Stability FoR to Body FoR/StabilityToBody ==
  note: body2wing
  note: Reshape creates array by arranging them in column first manner
  note: wing2stability
  note: wing2body
  note: stability2wing
  AoA : Inport
  Constant1 : Constant
  Constant{2..3,5..8,10..11} (8 alike) : Constant  Value=0
  Constant4 : Constant
  Cos1 : Trigonometry  Operator=cos
  Cos2 : Trigonometry  Operator=cos
  Gain1 : Gain  Gain=-1
  Gain2 : Gain  Gain=-1
  Matrix Multiply : Product  Multiplication=Matrix(*)
  Mux1 : Mux  Inputs=9
  Mux2 : Mux  Inputs=9
  Reshape1 : Reshape  OutputDimensionality=Customize  OutputDimensions=[3,3]
  Reshape2 : Reshape  OutputDimensionality=Customize  OutputDimensions=[3,3]
  Sin1 : Trigonometry
  Sin2 : Trigonometry
  Transpose : Math  Operator=transpose
  Transpose1 : Math  Operator=transpose
  body_wing_angle : Constant  Value=45*pi/180
  R_SB : Outport
  wires:
  Reshape2/1 -> Transpose/1
  AoA/1 -> Cos2/1, Sin2/1
  Sin2/1 -> [sinAoA]
  Mux2/1 -> Reshape2/1
  Cos2/1 -> [cosAoA]
  [sinAoA] -> Gain2/1
  [cosAoA] -> Mux2/1
  Constant2/1 -> Mux2/2
  [sinAoA] -> Mux2/3
  Constant3/1 -> Mux2/4
  Constant1/1 -> Mux2/5
  Constant10/1 -> Mux2/6
  Gain2/1 -> Mux2/7
  Constant11/1 -> Mux2/8
  [cosAoA] -> Mux2/9
  Transpose/1 -> Matrix Multiply/2
  Matrix Multiply/1 -> R_SB/1
  Constant5/1 -> Mux1/6
  [cosGamm] -> Mux1/1
  Constant8/1 -> Mux1/4
  Constant4/1 -> Mux1/5
  Constant6/1 -> Mux1/8
  [cosGamm] -> Mux1/9
  Constant7/1 -> Mux1/2
  Mux1/1 -> Reshape1/1
  Reshape1/1 -> Transpose1/1
  Transpose1/1 -> Matrix Multiply/1
  body_wing_angle/1 -> Sin1/1, Cos1/1
  Sin1/1 -> [sinGamm]
  Cos1/1 -> [cosGamm]
  [sinGamm] -> Gain1/1
  Gain1/1 -> Mux1/3
  [sinGamm] -> Mux1/7

== system test_8m_0508/Atmosphere_Model/EoM&Wind --> TAS/body2wing FoR ==
  u_body : Inport
  w_body : Inport  Port=2
  Add : Sum
  Add1 : Sum
  Cos2 : Trigonometry  Operator=cos
  Gain2 : Gain  Gain=-1
  Product{,1..3} (4 alike) : Product
  Sin2 : Trigonometry
  body_wing_angle : Constant  Value=45*pi/180
  u_wing : Outport
  w_wing : Outport  Port=2
  wires:
  Cos2/1 -> [cosGamm]
  Sin2/1 -> [sinGamm]
  [sinGamm] -> Gain2/1
  body_wing_angle/1 -> Sin2/1, Cos2/1
  [cosGamm] -> Product/2
  u_body/1 -> Product1/1, Product/1
  [sinGamm] -> Product1/2
  w_body/1 -> Product3/1, Product2/1
  Gain2/1 -> Product2/2
  [cosGamm] -> Product3/2
  Product/1 -> Add/1
  Product2/1 -> Add/2
  Product1/1 -> Add1/1
  Product3/1 -> Add1/2
  Add/1 -> u_wing/1
  Add1/1 -> w_wing/1

== system test_8m_0508/Atmosphere_Model/ISA_upto20km/Subsystem ==
  Th : Inport
  gamma : Inport  Port=2
  R : Inport  Port=3
  Product : Product
  Product1 : Product
  Sqrt : Sqrt
  Speed of Sound at h : Outport
  wires:
  R/1 -> Product/2
  Th/1 -> Product1/1
  Product1/1 -> Sqrt/1
  Sqrt/1 -> Speed of Sound at h/1
  Product/1 -> Product1/2
  gamma/1 -> Product/1

== system test_8m_0508/Atmosphere_Model/ISA_upto20km/Subsystem1 ==
  g0 : Inport
  a : Inport  Port=2
  R : Inport  Port=3
  T0 : Inport  Port=4
  h : Inport  Port=5
  P0 : Inport  Port=6
  rho0 : Inport  Port=7
  Add : Sum
  Add1 : Sum
  Add2 : Sum  Inputs=+-
  Constant : Constant  Value=-1
  Constant1 : Constant  Value=11000
  Display : Display
  Display1 : Display
  Divide : Product  Inputs=*/
  Divide1 : Product  Inputs=*/
  Divide2 : Product  Inputs=*/
  Gain : Gain  Gain=-1
  Gain1 : Gain  Gain=-1
  Power : Math  Operator=pow
  Power1 : Math  Operator=pow
  Power2 : Math
  Product{,1..7} (8 alike) : Product
  Saturation : Saturate  UpperLimit=11000  LowerLimit=0
  Saturation1 : Saturate  UpperLimit=25000  LowerLimit=11000
  Th : Outport
  Ph : Outport  Port=2
  rhoh : Outport  Port=3
  wires:
  Divide2/1 -> Power1/1, Power/1
  Divide1/1 -> Power/2, Add1/1  "-g/a*R"
  Product3/1 -> Product7/1
  Power/1 -> Product3/2
  Product2/1 -> Divide1/2
  Constant/1 -> Add1/2
  Gain/1 -> Divide1/1
  R/1 -> Product/1, Product2/2
  Power1/1 -> Product5/1
  rho0/1 -> Product5/2
  P0/1 -> Product3/1
  Add1/1 -> Power1/2
  g0/1 -> Gain1/1, Gain/1
  a/1 -> Product2/1, Product1/1
  Product5/1 -> Product6/1
  h/1 -> Saturation1/1, Saturation/1
  Product1/1 -> Add/1
  Add/1 -> Th/1, Product/2, Divide2/1  "Th"
  Saturation/1 -> Product1/2
  Saturation1/1 -> Add2/1
  Add2/1 -> Product4/1
  Constant1/1 -> Add2/2
  Product/1 -> Divide/2
  Divide/1 -> Product4/2
  Product4/1 -> Power2/1  "power"
  Power2/1 -> Display/1, Product6/2, Product7/2
  T0/1 -> Divide2/2, Add/2
  Gain1/1 -> Divide/1
  Product7/1 -> Ph/1
  Product6/1 -> Display1/1, rhoh/1

== system test_8m_0508/Atmosphere_Model/TAS2CAS/Subsystem ==
  ah : Inport
  TAS : Inport  Port=2
  Divide : Product  Inputs=*/
  Mach : Outport
  wires:
  ah/1 -> Divide/2
  Divide/1 -> Mach/1  "Mach"
  TAS/1 -> Divide/1

== system test_8m_0508/Atmosphere_Model/TAS2CAS/Subsystem1 ==
  In1 : Inport
  In2 : Inport  Port=2
  In3 : Inport  Port=3
  Product2 : Product
  Product3 : Product
  Sqrt : Sqrt
  a0 : Outport
  wires:
  Sqrt/1 -> a0/1  "a0"
  Product2/1 -> Product3/1
  Product3/1 -> Sqrt/1
  In1/1 -> Product2/1
  In3/1 -> Product3/2
  In2/1 -> Product2/2
